simulink model "Detumbling_using_engine_sim"  (R2022b)
settings: Solver=VariableStepAuto  StartTime=0.0  StopTime=Params.tf  FixedStep=1e-2  RelTol=1e-8  AbsTol=1e-8
values from neighbouring files (symbols this model uses):
  Pitch_thrust_operator = abs(-1/( (1/(norm(Params.arm_vec1)))*(sin(gamma1)*sin(theta)*Params.arm_vec1(3)-cos(gamma1)*Params.arm_vec1(1))+         (1/(norm(Params.arm_vec2)))*(-sin(gamma2)*sin(theta)*Params.arm_vec2(3)-cos(gamma2)*Params.arm_vec2(1))+         (1/(norm(Params.arm_vec3)))*(sin(gamma3)*cos(theta)*Params.arm_vec3(3)+cos(gamma3)*Params.arm_vec3(2))+         (1/(norm(Params.arm_vec4)))*(sin(gamma4)*sin(theta)*Pa ...(+61 chars)    [Detumbling_using_engine_SimCode.m]
  Roll_thrust_operator = abs(-1/( (1/(norm(Params.arm_vec1)))*(-sin(gamma1)*cos(theta)*Params.arm_vec1(3)+cos(gamma1)*Params.arm_vec1(2))+         (1/(norm(Params.arm_vec2)))*(-sin(gamma2)*cos(theta)*Params.arm_vec2(3)+cos(gamma2)*Params.arm_vec2(2))+         (1/(norm(Params.arm_vec3)))*(sin(gamma3)*sin(theta)*Params.arm_vec3(3)-cos(gamma3)*Params.arm_vec3(1))+         (1/(norm(Params.arm_vec4)))*(sin(gamma4)*cos(theta)*P ...(+51 chars)    [Detumbling_using_engine_SimCode.m]
  tau_Thrusters = 30e-03    (= 0.03)    [Detumbling_using_engine_SimCode.m]
  w_c = [0,0,0]'    [Detumbling_using_engine_SimCode.m]
  Yaw_thrust_operator = abs(-1/( (1/(norm(Params.arm_vec1)))*(-sin(gamma1)*sin(theta)*Params.arm_vec1(2)+cos(theta)*sin(gamma1)*Params.arm_vec1(1))+         (1/(norm(Params.arm_vec2)))*(-sin(gamma2)*sin(theta)*Params.arm_vec2(2)-cos(theta)*sin(gamma2)*Params.arm_vec2(1))+         (1/(norm(Params.arm_vec3)))*(-sin(gamma3)*sin(theta)*Params.arm_vec3(2)-sin(gamma3)*cos(theta)*Params.arm_vec3(1))+         (1/(norm(Params.arm ...(+86 chars)    [Detumbling_using_engine_SimCode.m]
undefined symbols (not defined in the file or in its folder): gain, Params, Pitch, rad, Roll, s, T1, time_T1, Yaw
libraries: matrix_library x24, aerolibconvert2 x1, simulink_extras x1, sharedutil x1
(part 2 of 2)

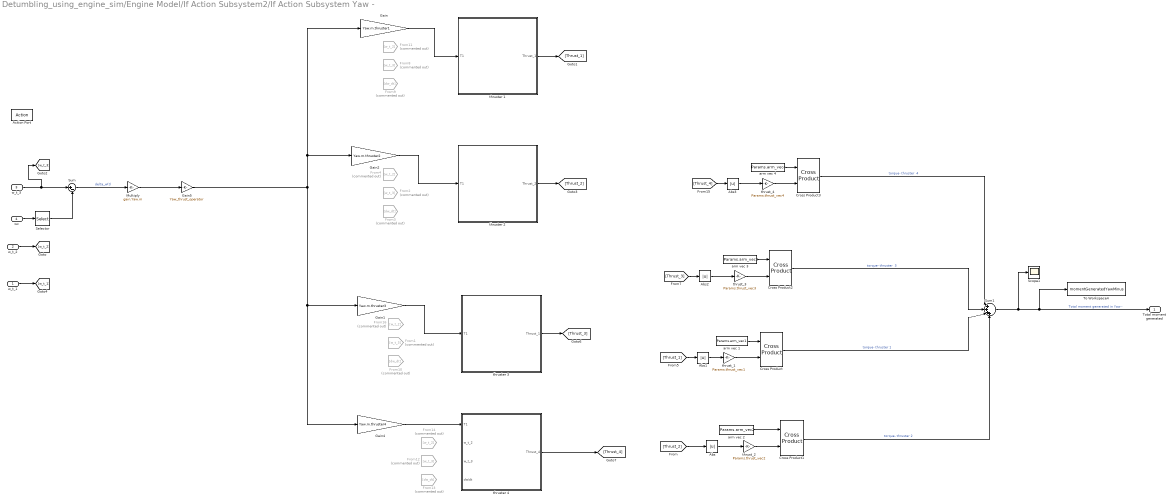
== system Detumbling_using_engine_sim/Engine Model/If Action Subsystem2/If Action Subsystem Yaw - ==
  w_t_1 : Inport
  w_t_2 : Inport  Port=2
  w_t_3 : Inport  Port=3
  wc : Inport  Port=4
  Action Port : ActionPort  ActionPortLabel=else
  Abs{,1..3} (4 alike) : Abs  SaturateOnIntegerOverflow=off
  Cross Product{,1..3} (4 alike) : matrix_library/Cross Product
  From{1..2,8,12} (4 alike) : From  Commented=on  GotoTag=w_t_3
  From{3,9..10,13} (4 alike) : From  Commented=on  GotoTag=dw_dt
  From{4,11,14,16} (4 alike) : From  Commented=on  GotoTag=w_t_2
  Gain : Gain  Gain=Yaw.m.thruster1
  Gain1 : Gain  Gain=Yaw.m.thruster3
  Gain2 : Gain  Gain=Yaw.m.thruster2
  Gain4 : Gain  Gain=Yaw.m.thruster4
  Gain5 : Gain  Gain=Yaw_thrust_operator
  Multiply : Gain  Gain=gain.Yaw.m
  Scope1 : Scope
  Selector : Selector  InputPortWidth=3  IndexOptions=Index vector (dialog)  Indices=3  OutputSizes=1
  Sum : Sum  Inputs=|+-
  Sum1 : Sum  Inputs=|++++
  To Workspace4 : ToWorkspace  VariableName=momentGeneratedYawMinus  SaveFormat=Timeseries  SampleTime=-1
  arm vec 1 : Constant  Value=Params.arm_vec1
  arm vec 2 : Constant  Value=Params.arm_vec2
  arm vec 3 : Constant  Value=Params.arm_vec3
  arm vec 4 : Constant  Value=Params.arm_vec4
  thrust_1 : Gain  Gain=Params.thrust_vec1
  thrust_2 : Gain  Gain=Params.thrust_vec2
  thrust_3 : Gain  Gain=Params.thrust_vec3
  thrust_4 : Gain  Gain=Params.thrust_vec4
  thruster 1 : Subsystem
  thruster 2 : Subsystem
  thruster 3 : Subsystem
  "thruster 4 " : Subsystem
  "Total moment generated " : Outport
  wires:
  w_t_1/1 -> [w_t_1]
  w_t_2/1 -> [w_t_2]
  w_t_3/1 -> [w_t_3], Sum/1
  wc/1 -> Selector/1
  Selector/1 -> Sum/2
  Multiply/1 -> Gain5/1
  thrust_3/1 -> Cross Product2/2
  Cross Product2/1 -> Sum1/2  "torque- thruster  3"
  Gain5/1 -> Gain2/1, Gain/1, Gain4/1, Gain1/1
  Cross Product3/1 -> Sum1/1  "torque- thruster  4"
  [Thrust_1] -> Abs1/1
  Gain/1 -> thruster 1/1(T1)
  Gain4/1 -> "thruster 4 "/1(T1)
  [Thrust_2] -> Abs/1
  arm vec 4/1 -> Cross Product3/1
  Cross Product/1 -> Sum1/3  "torque- thruster 1"
  thrust_4/1 -> Cross Product3/2
  arm vec 2/1 -> Cross Product1/1
  thruster 1/1(Thrust_1) -> [Thrust_1]
  arm vec 1/1 -> Cross Product/1
  thruster 3/1(Thrust_1) -> [Thrust_3]
  Cross Product1/1 -> Sum1/4  "torque- thruster 2"
  [Thrust_3] -> Abs2/1
  Gain2/1 -> thruster 2/1(T1)
  Sum/1 -> Multiply/1  "delta_w(t)"
  [Thrust_4] -> Abs3/1
  thrust_2/1 -> Cross Product1/2
  Abs1/1 -> thrust_1/1
  Sum1/1 -> Scope1/1, "Total moment generated "/1, To Workspace4/1  "Total moment generated in Yaw -"
  arm vec 3/1 -> Cross Product2/1
  Abs2/1 -> thrust_3/1
  "thruster 4 "/1(Thrust_4) -> [Thrust_4]
  Gain1/1 -> thruster 3/1(T1)
  Abs/1 -> thrust_2/1
  thruster 2/1(Thrust_2) -> [Thrust_2]
  Abs3/1 -> thrust_4/1
  thrust_1/1 -> Cross Product/2

== system Detumbling_using_engine_sim/Satellite Bus/Satellite Kinematics/CHI(q) ==
  q : Inport
  Demux : Demux
  Gain{1..6} (6 alike) : Gain  Gain=-1
  Vector Concatenate : Concatenate  NumInputs=4
  Vector Concatenate1 : Concatenate  NumInputs=4
  Vector Concatenate2 : Concatenate  NumInputs=4
  Vector Concatenate3 : Concatenate  NumInputs=3  Mode=Multidimensional array  ConcatenateDimension=2
  CHI : Outport
  wires:
  [q1] -> Vector Concatenate2/3
  [q3] -> Gain5/1
  Vector Concatenate3/1 -> CHI/1
  Vector Concatenate/1 -> Vector Concatenate3/1
  Vector Concatenate2/1 -> Vector Concatenate3/2
  q/1 -> Demux/1
  [q3] -> Gain3/1
  Gain3/1 -> Vector Concatenate2/1
  [q3] -> Vector Concatenate/2
  [q4] -> Vector Concatenate1/3
  [q1] -> Gain1/1
  Demux/2 -> [q2]
  Gain1/1 -> Vector Concatenate/4
  Demux/3 -> [q3]
  [q4] -> Vector Concatenate/1
  [q4] -> Vector Concatenate2/2
  Gain4/1 -> Vector Concatenate2/4
  [q2] -> Vector Concatenate1/1
  Demux/1 -> [q1]
  [q1] -> Gain6/1
  Gain6/1 -> Vector Concatenate1/2
  [q2] -> Gain2/1
  [q2] -> Gain4/1
  Gain2/1 -> Vector Concatenate/3
  Vector Concatenate1/1 -> Vector Concatenate3/3
  Demux/4 -> [q4]
  Gain5/1 -> Vector Concatenate1/4

== system Detumbling_using_engine_sim/Engine Model/If Action Subsystem/If Action Subsystem Roll +/thruster 1 ==
  T1 : Inport
  Abs : Abs  Commented=on  SaturateOnIntegerOverflow=off
  Clock : Clock  Commented=on
  Constant : Constant  Commented=on
  Divide : Product  Commented=on  Inputs=*/
  Divide1 : Product  Commented=on  Inputs=*/
  Divide2 : Product  Commented=on  Inputs=*/
  From{,1,3..4} (4 alike) : From  Commented=on  GotoTag=T1
  From2 : From  Commented=on  GotoTag=impulseBit_BiProp
  From5 : From  Commented=on  GotoTag=Stop_step
  Gain : Gain  Commented=on  Gain=Params.ImpulseBit_BiProp
  Goto2 : Goto  Commented=on  GotoTag=Stop_step
  Initial Body Angular rates [deg/sec] : Constant  Value=Params.ImpulseBit_BiProp
  Scope : Scope
  Step1 : Step  Commented=on  Time=Params.ImpulseBit_BiProp/T1  SampleTime=0
  Sum : Sum  Inputs=|+-
  Sum1 : Sum  Commented=on  Inputs=|++
  Switch : Switch  Commented=on  Criteria=u2 > Threshold  SaturateOnIntegerOverflow=off  InputSameDT=off
  "Time constant - open thruster " : TransferFcn  Denominator=[tau_Thrusters 1]
  To Workspace : ToWorkspace  Commented=on  VariableName=T1  SaveFormat=Timeseries  SampleTime=-1
  Variable Time Delay : VariableTransportDelay  Commented=on  MaximumDelay=50
  Thrust_1 : Outport
  wires:
  "Time constant - open thruster "/1 -> Sum/1
  Sum/1 -> Scope/1, Thrust_1/1
  Initial Body Angular rates [deg/sec]/1 -> [impulseBit_BiProp]
  Constant/1 -> Divide/1
  From/1 -> Divide/2
  Divide/1 -> Gain/1
  From1/1 -> Divide1/2
  Divide1/1 -> Sum1/2  "Requested Time [sec] The maximum possible"
  Clock/1 -> Sum1/1
  Sum1/1 -> Switch/2
  T1/1 -> [T1], To Workspace/1, "Time constant - open thruster "/1
  Divide2/1 -> Abs/1  "Maximum Time allowed"
  From2/1 -> Divide2/1
  From3/1 -> Divide2/2
  From4/1 -> Variable Time Delay/1
  Variable Time Delay/1 -> Goto2/1
  From5/1 -> Sum/2
  Abs/1 -> Variable Time Delay/2

== system Detumbling_using_engine_sim/Engine Model/If Action Subsystem/If Action Subsystem Roll +/thruster 2 ==
  T1 : Inport
  Abs : Abs  Commented=on  SaturateOnIntegerOverflow=off
  Divide2 : Product  Commented=on  Inputs=*/
  From2 : From  Commented=on  GotoTag=impulseBit_BiProp
  From3 : From  Commented=on  GotoTag=T2
  From4 : From  Commented=on  GotoTag=T2
  From5 : From  Commented=on  GotoTag=Stop_step
  Goto2 : Goto  Commented=on  GotoTag=Stop_step
  Initial Body Angular rates [deg/sec] : Constant  Value=Params.ImpulseBit_BiProp
  Scope : Scope
  Sum : Sum  Inputs=|+-
  "Time constant - open thruster " : TransferFcn  Denominator=[tau_Thrusters 1]
  To Workspace : ToWorkspace  Commented=on  VariableName=T1  SaveFormat=Timeseries  SampleTime=-1
  Variable Time Delay : VariableTransportDelay  Commented=on  MaximumDelay=50
  Thrust_2 : Outport
  wires:
  "Time constant - open thruster "/1 -> Sum/1
  Sum/1 -> Scope/1, Thrust_2/1
  Initial Body Angular rates [deg/sec]/1 -> [impulseBit_BiProp]
  T1/1 -> [T2], To Workspace/1, "Time constant - open thruster "/1
  From3/1 -> Divide2/2
  Divide2/1 -> Abs/1  "Maximum Time allowed"
  From4/1 -> Variable Time Delay/1
  Variable Time Delay/1 -> Goto2/1
  From2/1 -> Divide2/1
  From5/1 -> Sum/2
  Abs/1 -> Variable Time Delay/2

== system Detumbling_using_engine_sim/Engine Model/If Action Subsystem/If Action Subsystem Roll +/thruster 3 ==
  T1 : Inport
  Abs : Abs  Commented=on  SaturateOnIntegerOverflow=off
  Divide2 : Product  Commented=on  Inputs=*/
  From2 : From  Commented=on  GotoTag=impulseBit_BiProp
  From3 : From  Commented=on  GotoTag=T3
  From4 : From  Commented=on  GotoTag=T3
  From5 : From  Commented=on  GotoTag=Stop_step
  Goto2 : Goto  Commented=on  GotoTag=Stop_step
  Initial Body Angular rates [deg/sec] : Constant  Value=Params.ImpulseBit_BiProp
  Scope : Scope
  Sum : Sum  Inputs=|+-
  "Time constant - open thruster " : TransferFcn  Denominator=[tau_Thrusters 1]
  To Workspace : ToWorkspace  Commented=on  VariableName=T1  SaveFormat=Timeseries  SampleTime=-1
  Variable Time Delay1 : VariableTransportDelay  Commented=on  MaximumDelay=50
  Thrust_1 : Outport
  wires:
  "Time constant - open thruster "/1 -> Sum/1
  Sum/1 -> Scope/1, Thrust_1/1
  Initial Body Angular rates [deg/sec]/1 -> [impulseBit_BiProp]
  T1/1 -> [T3], To Workspace/1, "Time constant - open thruster "/1
  From3/1 -> Divide2/2
  Divide2/1 -> Abs/1  "Maximum Time allowed"
  From4/1 -> Variable Time Delay1/1
  Variable Time Delay1/1 -> Goto2/1
  From2/1 -> Divide2/1
  From5/1 -> Sum/2
  Abs/1 -> Variable Time Delay1/2

== system Detumbling_using_engine_sim/Engine Model/If Action Subsystem/If Action Subsystem Roll +/thruster 4  ==
  T1 : Inport
  w_t_2 : Inport  Port=2
  w_t_3 : Inport  Port=3
  dw/dt : Inport  Port=4
  Abs : Abs  Commented=on  SaturateOnIntegerOverflow=off
  Divide2 : Product  Commented=on  Inputs=*/
  From2 : From  Commented=on  GotoTag=impulseBit_BiProp
  From3 : From  Commented=on  GotoTag=T1
  From4 : From  Commented=on  GotoTag=T1
  From5 : From  Commented=on  GotoTag=Stop_step
  Goto2 : Goto  Commented=on  GotoTag=Stop_step
  Initial Body Angular rates [deg/sec] : Constant  Value=Params.ImpulseBit_BiProp
  Sum : Sum  Inputs=|+-
  "Time constant - open thruster " : TransferFcn  Denominator=[tau_Thrusters 1]
  To Workspace : ToWorkspace  Commented=on  VariableName=T1  SaveFormat=Timeseries  SampleTime=-1
  Variable Time Delay1 : VariableTransportDelay  Commented=on  MaximumDelay=50
  Thrust_4 : Outport
  wires:
  "Time constant - open thruster "/1 -> Sum/1
  Sum/1 -> Thrust_4/1
  Initial Body Angular rates [deg/sec]/1 -> [impulseBit_BiProp]
  T1/1 -> [T1], To Workspace/1, "Time constant - open thruster "/1
  From2/1 -> Divide2/1
  From3/1 -> Divide2/2
  Divide2/1 -> Abs/1  "Maximum Time allowed"
  From4/1 -> Variable Time Delay1/1
  Variable Time Delay1/1 -> Goto2/1
  From5/1 -> Sum/2
  Abs/1 -> Variable Time Delay1/2

== system Detumbling_using_engine_sim/Engine Model/If Action Subsystem/If Action Subsystem Roll -/thruster 1 ==
  T1 : Inport
  Abs : Abs  Commented=on  SaturateOnIntegerOverflow=off
  Clock : Clock  Commented=on
  Constant : Constant  Commented=on
  Divide : Product  Commented=on  Inputs=*/
  Divide1 : Product  Commented=on  Inputs=*/
  Divide2 : Product  Commented=on  Inputs=*/
  From{,1,3..4} (4 alike) : From  Commented=on  GotoTag=T1
  From2 : From  Commented=on  GotoTag=impulseBit_BiProp
  From5 : From  Commented=on  GotoTag=Stop_step
  Gain : Gain  Commented=on  Gain=Params.ImpulseBit_BiProp
  Goto2 : Goto  Commented=on  GotoTag=Stop_step
  Initial Body Angular rates [deg/sec] : Constant  Value=Params.ImpulseBit_BiProp
  Scope : Scope
  Step1 : Step  Commented=on  Time=Params.ImpulseBit_BiProp/T1  SampleTime=0
  Sum : Sum  Inputs=|+-
  Sum1 : Sum  Commented=on  Inputs=|++
  Switch : Switch  Commented=on  Criteria=u2 > Threshold  SaturateOnIntegerOverflow=off  InputSameDT=off
  "Time constant - open thruster " : TransferFcn  Denominator=[tau_Thrusters 1]
  To Workspace : ToWorkspace  Commented=on  VariableName=T1  SaveFormat=Timeseries  SampleTime=-1
  Variable Time Delay : VariableTransportDelay  Commented=on  MaximumDelay=50
  Thrust_1 : Outport
  wires:
  "Time constant - open thruster "/1 -> Sum/1
  Sum/1 -> Scope/1, Thrust_1/1
  Initial Body Angular rates [deg/sec]/1 -> [impulseBit_BiProp]
  Constant/1 -> Divide/1
  From/1 -> Divide/2
  Divide/1 -> Gain/1
  From1/1 -> Divide1/2
  Divide1/1 -> Sum1/2  "Requested Time [sec] The maximum possible"
  Clock/1 -> Sum1/1
  Sum1/1 -> Switch/2
  T1/1 -> [T1], To Workspace/1, "Time constant - open thruster "/1
  Divide2/1 -> Abs/1  "Maximum Time allowed"
  From2/1 -> Divide2/1
  From3/1 -> Divide2/2
  From4/1 -> Variable Time Delay/1
  Variable Time Delay/1 -> Goto2/1
  From5/1 -> Sum/2
  Abs/1 -> Variable Time Delay/2

== system Detumbling_using_engine_sim/Engine Model/If Action Subsystem/If Action Subsystem Roll -/thruster 2 ==
  T1 : Inport
  Abs : Abs  Commented=on  SaturateOnIntegerOverflow=off
  Divide2 : Product  Commented=on  Inputs=*/
  From2 : From  Commented=on  GotoTag=impulseBit_BiProp
  From3 : From  Commented=on  GotoTag=T2
  From4 : From  Commented=on  GotoTag=T2
  From5 : From  Commented=on  GotoTag=Stop_step
  Goto2 : Goto  Commented=on  GotoTag=Stop_step
  Initial Body Angular rates [deg/sec] : Constant  Value=Params.ImpulseBit_BiProp
  Scope : Scope
  Sum : Sum  Inputs=|+-
  "Time constant - open thruster " : TransferFcn  Denominator=[tau_Thrusters 1]
  To Workspace : ToWorkspace  Commented=on  VariableName=T1  SaveFormat=Timeseries  SampleTime=-1
  Variable Time Delay : VariableTransportDelay  Commented=on  MaximumDelay=50
  Thrust_2 : Outport
  wires:
  "Time constant - open thruster "/1 -> Sum/1
  Sum/1 -> Scope/1, Thrust_2/1
  Initial Body Angular rates [deg/sec]/1 -> [impulseBit_BiProp]
  T1/1 -> [T2], To Workspace/1, "Time constant - open thruster "/1
  From3/1 -> Divide2/2
  Divide2/1 -> Abs/1  "Maximum Time allowed"
  From4/1 -> Variable Time Delay/1
  Variable Time Delay/1 -> Goto2/1
  From2/1 -> Divide2/1
  From5/1 -> Sum/2
  Abs/1 -> Variable Time Delay/2

== system Detumbling_using_engine_sim/Engine Model/If Action Subsystem/If Action Subsystem Roll -/thruster 3 ==
  T1 : Inport
  Abs : Abs  Commented=on  SaturateOnIntegerOverflow=off
  Divide2 : Product  Commented=on  Inputs=*/
  From2 : From  Commented=on  GotoTag=impulseBit_BiProp
  From3 : From  Commented=on  GotoTag=T3
  From4 : From  Commented=on  GotoTag=T3
  From5 : From  Commented=on  GotoTag=Stop_step
  Goto2 : Goto  Commented=on  GotoTag=Stop_step
  Initial Body Angular rates [deg/sec] : Constant  Value=Params.ImpulseBit_BiProp
  Scope : Scope
  Sum : Sum  Inputs=|+-
  "Time constant - open thruster " : TransferFcn  Denominator=[tau_Thrusters 1]
  To Workspace : ToWorkspace  Commented=on  VariableName=T1  SaveFormat=Timeseries  SampleTime=-1
  Variable Time Delay1 : VariableTransportDelay  Commented=on  MaximumDelay=50
  Thrust_1 : Outport
  wires:
  "Time constant - open thruster "/1 -> Sum/1
  Sum/1 -> Scope/1, Thrust_1/1
  Initial Body Angular rates [deg/sec]/1 -> [impulseBit_BiProp]
  T1/1 -> [T3], To Workspace/1, "Time constant - open thruster "/1
  From3/1 -> Divide2/2
  Divide2/1 -> Abs/1  "Maximum Time allowed"
  From4/1 -> Variable Time Delay1/1
  Variable Time Delay1/1 -> Goto2/1
  From2/1 -> Divide2/1
  From5/1 -> Sum/2
  Abs/1 -> Variable Time Delay1/2

== system Detumbling_using_engine_sim/Engine Model/If Action Subsystem/If Action Subsystem Roll -/thruster 4  ==
  T1 : Inport
  w_t_2 : Inport  Port=2
  w_t_3 : Inport  Port=3
  dw/dt : Inport  Port=4
  Abs : Abs  Commented=on  SaturateOnIntegerOverflow=off
  Divide2 : Product  Commented=on  Inputs=*/
  From2 : From  Commented=on  GotoTag=impulseBit_BiProp
  From3 : From  Commented=on  GotoTag=T1
  From4 : From  Commented=on  GotoTag=T1
  From5 : From  Commented=on  GotoTag=Stop_step
  Goto2 : Goto  Commented=on  GotoTag=Stop_step
  Initial Body Angular rates [deg/sec] : Constant  Value=Params.ImpulseBit_BiProp
  Sum : Sum  Inputs=|+-
  "Time constant - open thruster " : TransferFcn  Denominator=[tau_Thrusters 1]
  To Workspace : ToWorkspace  Commented=on  VariableName=T1  SaveFormat=Timeseries  SampleTime=-1
  Variable Time Delay1 : VariableTransportDelay  Commented=on  MaximumDelay=50
  Thrust_4 : Outport
  wires:
  "Time constant - open thruster "/1 -> Sum/1
  Sum/1 -> Thrust_4/1
  Initial Body Angular rates [deg/sec]/1 -> [impulseBit_BiProp]
  T1/1 -> [T1], To Workspace/1, "Time constant - open thruster "/1
  From2/1 -> Divide2/1
  From3/1 -> Divide2/2
  Divide2/1 -> Abs/1  "Maximum Time allowed"
  From4/1 -> Variable Time Delay1/1
  Variable Time Delay1/1 -> Goto2/1
  From5/1 -> Sum/2
  Abs/1 -> Variable Time Delay1/2

== system Detumbling_using_engine_sim/Engine Model/If Action Subsystem1/If Action Subsystem Pitch +/thruster 1 ==
  T1 : Inport
  Abs : Abs  Commented=on  SaturateOnIntegerOverflow=off
  Clock : Clock  Commented=on
  Constant : Constant  Commented=on
  Divide : Product  Commented=on  Inputs=*/
  Divide1 : Product  Commented=on  Inputs=*/
  Divide2 : Product  Commented=on  Inputs=*/
  From{,1,3..4} (4 alike) : From  Commented=on  GotoTag=T1
  From2 : From  Commented=on  GotoTag=impulseBit_BiProp
  From5 : From  Commented=on  GotoTag=Stop_step
  Gain : Gain  Commented=on  Gain=Params.ImpulseBit_BiProp
  Goto2 : Goto  Commented=on  GotoTag=Stop_step
  Initial Body Angular rates [deg/sec] : Constant  Value=Params.ImpulseBit_BiProp
  Scope : Scope
  Step1 : Step  Commented=on  Time=Params.ImpulseBit_BiProp/T1  SampleTime=0
  Sum : Sum  Inputs=|+-
  Sum1 : Sum  Commented=on  Inputs=|++
  Switch : Switch  Commented=on  Criteria=u2 > Threshold  SaturateOnIntegerOverflow=off  InputSameDT=off
  "Time constant - open thruster " : TransferFcn  Denominator=[tau_Thrusters 1]
  To Workspace : ToWorkspace  Commented=on  VariableName=T1  SaveFormat=Timeseries  SampleTime=-1
  Variable Time Delay : VariableTransportDelay  Commented=on  MaximumDelay=50
  Thrust_1 : Outport
  wires:
  "Time constant - open thruster "/1 -> Sum/1
  Sum/1 -> Scope/1, Thrust_1/1
  Initial Body Angular rates [deg/sec]/1 -> [impulseBit_BiProp]
  Constant/1 -> Divide/1
  From/1 -> Divide/2
  Divide/1 -> Gain/1
  From1/1 -> Divide1/2
  Divide1/1 -> Sum1/2  "Requested Time [sec] The maximum possible"
  Clock/1 -> Sum1/1
  Sum1/1 -> Switch/2
  T1/1 -> [T1], To Workspace/1, "Time constant - open thruster "/1
  Divide2/1 -> Abs/1  "Maximum Time allowed"
  From2/1 -> Divide2/1
  From3/1 -> Divide2/2
  From4/1 -> Variable Time Delay/1
  Variable Time Delay/1 -> Goto2/1
  From5/1 -> Sum/2
  Abs/1 -> Variable Time Delay/2

== system Detumbling_using_engine_sim/Engine Model/If Action Subsystem1/If Action Subsystem Pitch +/thruster 2 ==
  T1 : Inport
  Abs : Abs  Commented=on  SaturateOnIntegerOverflow=off
  Divide2 : Product  Commented=on  Inputs=*/
  From2 : From  Commented=on  GotoTag=impulseBit_BiProp
  From3 : From  Commented=on  GotoTag=T2
  From4 : From  Commented=on  GotoTag=T2
  From5 : From  Commented=on  GotoTag=Stop_step
  Goto2 : Goto  Commented=on  GotoTag=Stop_step
  Initial Body Angular rates [deg/sec] : Constant  Value=Params.ImpulseBit_BiProp
  Scope : Scope
  Sum : Sum  Inputs=|+-
  "Time constant - open thruster " : TransferFcn  Denominator=[tau_Thrusters 1]
  To Workspace : ToWorkspace  Commented=on  VariableName=T1  SaveFormat=Timeseries  SampleTime=-1
  Variable Time Delay : VariableTransportDelay  Commented=on  MaximumDelay=50
  Thrust_2 : Outport
  wires:
  "Time constant - open thruster "/1 -> Sum/1
  Sum/1 -> Scope/1, Thrust_2/1
  Initial Body Angular rates [deg/sec]/1 -> [impulseBit_BiProp]
  T1/1 -> [T2], To Workspace/1, "Time constant - open thruster "/1
  From3/1 -> Divide2/2
  Divide2/1 -> Abs/1  "Maximum Time allowed"
  From4/1 -> Variable Time Delay/1
  Variable Time Delay/1 -> Goto2/1
  From2/1 -> Divide2/1
  From5/1 -> Sum/2
  Abs/1 -> Variable Time Delay/2

== system Detumbling_using_engine_sim/Engine Model/If Action Subsystem1/If Action Subsystem Pitch +/thruster 3 ==
  T1 : Inport
  Abs : Abs  Commented=on  SaturateOnIntegerOverflow=off
  Divide2 : Product  Commented=on  Inputs=*/
  From2 : From  Commented=on  GotoTag=impulseBit_BiProp
  From3 : From  Commented=on  GotoTag=T3
  From4 : From  Commented=on  GotoTag=T3
  From5 : From  Commented=on  GotoTag=Stop_step
  Goto2 : Goto  Commented=on  GotoTag=Stop_step
  Initial Body Angular rates [deg/sec] : Constant  Value=Params.ImpulseBit_BiProp
  Scope : Scope
  Sum : Sum  Inputs=|+-
  "Time constant - open thruster " : TransferFcn  Denominator=[tau_Thrusters 1]
  To Workspace : ToWorkspace  Commented=on  VariableName=T1  SaveFormat=Timeseries  SampleTime=-1
  Variable Time Delay1 : VariableTransportDelay  Commented=on  MaximumDelay=50
  Thrust_1 : Outport
  wires:
  "Time constant - open thruster "/1 -> Sum/1
  Sum/1 -> Scope/1, Thrust_1/1
  Initial Body Angular rates [deg/sec]/1 -> [impulseBit_BiProp]
  T1/1 -> [T3], To Workspace/1, "Time constant - open thruster "/1
  From3/1 -> Divide2/2
  Divide2/1 -> Abs/1  "Maximum Time allowed"
  From4/1 -> Variable Time Delay1/1
  Variable Time Delay1/1 -> Goto2/1
  From2/1 -> Divide2/1
  From5/1 -> Sum/2
  Abs/1 -> Variable Time Delay1/2

== system Detumbling_using_engine_sim/Engine Model/If Action Subsystem1/If Action Subsystem Pitch +/thruster 4  ==
  T1 : Inport
  w_t_2 : Inport  Port=2
  w_t_3 : Inport  Port=3
  dw/dt : Inport  Port=4
  Abs : Abs  Commented=on  SaturateOnIntegerOverflow=off
  Divide2 : Product  Commented=on  Inputs=*/
  From2 : From  Commented=on  GotoTag=impulseBit_BiProp
  From3 : From  Commented=on  GotoTag=T1
  From4 : From  Commented=on  GotoTag=T1
  From5 : From  Commented=on  GotoTag=Stop_step
  Goto2 : Goto  Commented=on  GotoTag=Stop_step
  Initial Body Angular rates [deg/sec] : Constant  Value=Params.ImpulseBit_BiProp
  Sum : Sum  Inputs=|+-
  "Time constant - open thruster " : TransferFcn  Denominator=[tau_Thrusters 1]
  To Workspace : ToWorkspace  Commented=on  VariableName=T1  SaveFormat=Timeseries  SampleTime=-1
  Variable Time Delay1 : VariableTransportDelay  Commented=on  MaximumDelay=50
  Thrust_4 : Outport
  wires:
  "Time constant - open thruster "/1 -> Sum/1
  Sum/1 -> Thrust_4/1
  Initial Body Angular rates [deg/sec]/1 -> [impulseBit_BiProp]
  T1/1 -> [T1], To Workspace/1, "Time constant - open thruster "/1
  From2/1 -> Divide2/1
  From3/1 -> Divide2/2
  Divide2/1 -> Abs/1  "Maximum Time allowed"
  From4/1 -> Variable Time Delay1/1
  Variable Time Delay1/1 -> Goto2/1
  From5/1 -> Sum/2
  Abs/1 -> Variable Time Delay1/2

== system Detumbling_using_engine_sim/Engine Model/If Action Subsystem1/If Action Subsystem Pitch -/thruster 1 ==
  T1 : Inport
  Abs : Abs  Commented=on  SaturateOnIntegerOverflow=off
  Clock : Clock  Commented=on
  Constant : Constant  Commented=on
  Divide : Product  Commented=on  Inputs=*/
  Divide1 : Product  Commented=on  Inputs=*/
  Divide2 : Product  Commented=on  Inputs=*/
  From{,1,3..4} (4 alike) : From  Commented=on  GotoTag=T1
  From2 : From  Commented=on  GotoTag=impulseBit_BiProp
  From5 : From  Commented=on  GotoTag=Stop_step
  Gain : Gain  Commented=on  Gain=Params.ImpulseBit_BiProp
  Goto2 : Goto  Commented=on  GotoTag=Stop_step
  Initial Body Angular rates [deg/sec] : Constant  Value=Params.ImpulseBit_BiProp
  Scope : Scope
  Step1 : Step  Commented=on  Time=Params.ImpulseBit_BiProp/T1  SampleTime=0
  Sum : Sum  Inputs=|+-
  Sum1 : Sum  Commented=on  Inputs=|++
  Switch : Switch  Commented=on  Criteria=u2 > Threshold  SaturateOnIntegerOverflow=off  InputSameDT=off
  "Time constant - open thruster " : TransferFcn  Denominator=[tau_Thrusters 1]
  To Workspace : ToWorkspace  Commented=on  VariableName=T1  SaveFormat=Timeseries  SampleTime=-1
  Variable Time Delay : VariableTransportDelay  Commented=on  MaximumDelay=50
  Thrust_1 : Outport
  wires:
  "Time constant - open thruster "/1 -> Sum/1
  Sum/1 -> Scope/1, Thrust_1/1
  Initial Body Angular rates [deg/sec]/1 -> [impulseBit_BiProp]
  Constant/1 -> Divide/1
  From/1 -> Divide/2
  Divide/1 -> Gain/1
  From1/1 -> Divide1/2
  Divide1/1 -> Sum1/2  "Requested Time [sec] The maximum possible"
  Clock/1 -> Sum1/1
  Sum1/1 -> Switch/2
  T1/1 -> [T1], To Workspace/1, "Time constant - open thruster "/1
  Divide2/1 -> Abs/1  "Maximum Time allowed"
  From2/1 -> Divide2/1
  From3/1 -> Divide2/2
  From4/1 -> Variable Time Delay/1
  Variable Time Delay/1 -> Goto2/1
  From5/1 -> Sum/2
  Abs/1 -> Variable Time Delay/2

== system Detumbling_using_engine_sim/Engine Model/If Action Subsystem1/If Action Subsystem Pitch -/thruster 2 ==
  T1 : Inport
  Abs : Abs  Commented=on  SaturateOnIntegerOverflow=off
  Divide2 : Product  Commented=on  Inputs=*/
  From2 : From  Commented=on  GotoTag=impulseBit_BiProp
  From3 : From  Commented=on  GotoTag=T2
  From4 : From  Commented=on  GotoTag=T2
  From5 : From  Commented=on  GotoTag=Stop_step
  Goto2 : Goto  Commented=on  GotoTag=Stop_step
  Initial Body Angular rates [deg/sec] : Constant  Value=Params.ImpulseBit_BiProp
  Scope : Scope
  Sum : Sum  Inputs=|+-
  "Time constant - open thruster " : TransferFcn  Denominator=[tau_Thrusters 1]
  To Workspace : ToWorkspace  Commented=on  VariableName=T1  SaveFormat=Timeseries  SampleTime=-1
  Variable Time Delay : VariableTransportDelay  Commented=on  MaximumDelay=50
  Thrust_2 : Outport
  wires:
  "Time constant - open thruster "/1 -> Sum/1
  Sum/1 -> Scope/1, Thrust_2/1
  Initial Body Angular rates [deg/sec]/1 -> [impulseBit_BiProp]
  T1/1 -> [T2], To Workspace/1, "Time constant - open thruster "/1
  From3/1 -> Divide2/2
  Divide2/1 -> Abs/1  "Maximum Time allowed"
  From4/1 -> Variable Time Delay/1
  Variable Time Delay/1 -> Goto2/1
  From2/1 -> Divide2/1
  From5/1 -> Sum/2
  Abs/1 -> Variable Time Delay/2

== system Detumbling_using_engine_sim/Engine Model/If Action Subsystem1/If Action Subsystem Pitch -/thruster 3 ==
  T1 : Inport
  Abs : Abs  Commented=on  SaturateOnIntegerOverflow=off
  Divide2 : Product  Commented=on  Inputs=*/
  From2 : From  Commented=on  GotoTag=impulseBit_BiProp
  From3 : From  Commented=on  GotoTag=T3
  From4 : From  Commented=on  GotoTag=T3
  From5 : From  Commented=on  GotoTag=Stop_step
  Goto2 : Goto  Commented=on  GotoTag=Stop_step
  Initial Body Angular rates [deg/sec] : Constant  Value=Params.ImpulseBit_BiProp
  Scope : Scope
  Sum : Sum  Inputs=|+-
  "Time constant - open thruster " : TransferFcn  Denominator=[tau_Thrusters 1]
  To Workspace : ToWorkspace  Commented=on  VariableName=T1  SaveFormat=Timeseries  SampleTime=-1
  Variable Time Delay1 : VariableTransportDelay  Commented=on  MaximumDelay=50
  Thrust_1 : Outport
  wires:
  "Time constant - open thruster "/1 -> Sum/1
  Sum/1 -> Scope/1, Thrust_1/1
  Initial Body Angular rates [deg/sec]/1 -> [impulseBit_BiProp]
  T1/1 -> [T3], To Workspace/1, "Time constant - open thruster "/1
  From3/1 -> Divide2/2
  Divide2/1 -> Abs/1  "Maximum Time allowed"
  From4/1 -> Variable Time Delay1/1
  Variable Time Delay1/1 -> Goto2/1
  From2/1 -> Divide2/1
  From5/1 -> Sum/2
  Abs/1 -> Variable Time Delay1/2

== system Detumbling_using_engine_sim/Engine Model/If Action Subsystem1/If Action Subsystem Pitch -/thruster 4  ==
  T1 : Inport
  w_t_2 : Inport  Port=2
  w_t_3 : Inport  Port=3
  dw/dt : Inport  Port=4
  Abs : Abs  Commented=on  SaturateOnIntegerOverflow=off
  Divide2 : Product  Commented=on  Inputs=*/
  From2 : From  Commented=on  GotoTag=impulseBit_BiProp
  From3 : From  Commented=on  GotoTag=T1
  From4 : From  Commented=on  GotoTag=T1
  From5 : From  Commented=on  GotoTag=Stop_step
  Goto2 : Goto  Commented=on  GotoTag=Stop_step
  Initial Body Angular rates [deg/sec] : Constant  Value=Params.ImpulseBit_BiProp
  Sum : Sum  Inputs=|+-
  "Time constant - open thruster " : TransferFcn  Denominator=[tau_Thrusters 1]
  To Workspace : ToWorkspace  Commented=on  VariableName=T1  SaveFormat=Timeseries  SampleTime=-1
  Variable Time Delay1 : VariableTransportDelay  Commented=on  MaximumDelay=50
  Thrust_4 : Outport
  wires:
  "Time constant - open thruster "/1 -> Sum/1
  Sum/1 -> Thrust_4/1
  Initial Body Angular rates [deg/sec]/1 -> [impulseBit_BiProp]
  T1/1 -> [T1], To Workspace/1, "Time constant - open thruster "/1
  From2/1 -> Divide2/1
  From3/1 -> Divide2/2
  Divide2/1 -> Abs/1  "Maximum Time allowed"
  From4/1 -> Variable Time Delay1/1
  Variable Time Delay1/1 -> Goto2/1
  From5/1 -> Sum/2
  Abs/1 -> Variable Time Delay1/2

== system Detumbling_using_engine_sim/Engine Model/If Action Subsystem2/If Action Subsystem Yaw +/thruster 1 ==
  T1 : Inport
  Abs : Abs  Commented=on  SaturateOnIntegerOverflow=off
  Clock : Clock  Commented=on
  Constant : Constant  Commented=on
  Divide : Product  Commented=on  Inputs=*/
  Divide1 : Product  Commented=on  Inputs=*/
  Divide2 : Product  Commented=on  Inputs=*/
  From{,1,3..4} (4 alike) : From  Commented=on  GotoTag=T1
  From2 : From  Commented=on  GotoTag=impulseBit_BiProp
  From5 : From  Commented=on  GotoTag=Stop_step
  Gain : Gain  Commented=on  Gain=Params.ImpulseBit_BiProp
  Goto2 : Goto  Commented=on  GotoTag=Stop_step
  Initial Body Angular rates [deg/sec] : Constant  Value=Params.ImpulseBit_BiProp
  Scope : Scope
  Step1 : Step  Commented=on  Time=Params.ImpulseBit_BiProp/T1  SampleTime=0
  Sum : Sum  Inputs=|+-
  Sum1 : Sum  Commented=on  Inputs=|++
  Switch : Switch  Commented=on  Criteria=u2 > Threshold  SaturateOnIntegerOverflow=off  InputSameDT=off
  "Time constant - open thruster " : TransferFcn  Denominator=[tau_Thrusters 1]
  To Workspace : ToWorkspace  Commented=on  VariableName=T1  SaveFormat=Timeseries  SampleTime=-1
  Variable Time Delay : VariableTransportDelay  Commented=on  MaximumDelay=50
  Thrust_1 : Outport
  wires:
  "Time constant - open thruster "/1 -> Sum/1
  Sum/1 -> Scope/1, Thrust_1/1
  Initial Body Angular rates [deg/sec]/1 -> [impulseBit_BiProp]
  Constant/1 -> Divide/1
  From/1 -> Divide/2
  Divide/1 -> Gain/1
  From1/1 -> Divide1/2
  Divide1/1 -> Sum1/2  "Requested Time [sec] The maximum possible"
  Clock/1 -> Sum1/1
  Sum1/1 -> Switch/2
  T1/1 -> [T1], To Workspace/1, "Time constant - open thruster "/1
  Divide2/1 -> Abs/1  "Maximum Time allowed"
  From2/1 -> Divide2/1
  From3/1 -> Divide2/2
  From4/1 -> Variable Time Delay/1
  Variable Time Delay/1 -> Goto2/1
  From5/1 -> Sum/2
  Abs/1 -> Variable Time Delay/2

== system Detumbling_using_engine_sim/Engine Model/If Action Subsystem2/If Action Subsystem Yaw +/thruster 2 ==
  T1 : Inport
  Abs : Abs  Commented=on  SaturateOnIntegerOverflow=off
  Divide2 : Product  Commented=on  Inputs=*/
  From2 : From  Commented=on  GotoTag=impulseBit_BiProp
  From3 : From  Commented=on  GotoTag=T2
  From4 : From  Commented=on  GotoTag=T2
  From5 : From  Commented=on  GotoTag=Stop_step
  Goto2 : Goto  Commented=on  GotoTag=Stop_step
  Initial Body Angular rates [deg/sec] : Constant  Value=Params.ImpulseBit_BiProp
  Scope : Scope
  Sum : Sum  Inputs=|+-
  "Time constant - open thruster " : TransferFcn  Denominator=[tau_Thrusters 1]
  To Workspace : ToWorkspace  Commented=on  VariableName=T1  SaveFormat=Timeseries  SampleTime=-1
  Variable Time Delay : VariableTransportDelay  Commented=on  MaximumDelay=50
  Thrust_2 : Outport
  wires:
  "Time constant - open thruster "/1 -> Sum/1
  Sum/1 -> Scope/1, Thrust_2/1
  Initial Body Angular rates [deg/sec]/1 -> [impulseBit_BiProp]
  T1/1 -> [T2], To Workspace/1, "Time constant - open thruster "/1
  From3/1 -> Divide2/2
  Divide2/1 -> Abs/1  "Maximum Time allowed"
  From4/1 -> Variable Time Delay/1
  Variable Time Delay/1 -> Goto2/1
  From2/1 -> Divide2/1
  From5/1 -> Sum/2
  Abs/1 -> Variable Time Delay/2

== system Detumbling_using_engine_sim/Engine Model/If Action Subsystem2/If Action Subsystem Yaw +/thruster 3 ==
  T1 : Inport
  Abs : Abs  Commented=on  SaturateOnIntegerOverflow=off
  Divide2 : Product  Commented=on  Inputs=*/
  From2 : From  Commented=on  GotoTag=impulseBit_BiProp
  From3 : From  Commented=on  GotoTag=T3
  From4 : From  Commented=on  GotoTag=T3
  From5 : From  Commented=on  GotoTag=Stop_step
  Goto2 : Goto  Commented=on  GotoTag=Stop_step
  Initial Body Angular rates [deg/sec] : Constant  Value=Params.ImpulseBit_BiProp
  Scope : Scope
  Sum : Sum  Inputs=|+-
  "Time constant - open thruster " : TransferFcn  Denominator=[tau_Thrusters 1]
  To Workspace : ToWorkspace  Commented=on  VariableName=T1  SaveFormat=Timeseries  SampleTime=-1
  Variable Time Delay1 : VariableTransportDelay  Commented=on  MaximumDelay=50
  Thrust_1 : Outport
  wires:
  "Time constant - open thruster "/1 -> Sum/1
  Sum/1 -> Scope/1, Thrust_1/1
  Initial Body Angular rates [deg/sec]/1 -> [impulseBit_BiProp]
  T1/1 -> [T3], To Workspace/1, "Time constant - open thruster "/1
  From3/1 -> Divide2/2
  Divide2/1 -> Abs/1  "Maximum Time allowed"
  From4/1 -> Variable Time Delay1/1
  Variable Time Delay1/1 -> Goto2/1
  From2/1 -> Divide2/1
  From5/1 -> Sum/2
  Abs/1 -> Variable Time Delay1/2

== system Detumbling_using_engine_sim/Engine Model/If Action Subsystem2/If Action Subsystem Yaw +/thruster 4  ==
  T1 : Inport
  w_t_2 : Inport  Port=2
  w_t_3 : Inport  Port=3
  dw/dt : Inport  Port=4
  Abs : Abs  Commented=on  SaturateOnIntegerOverflow=off
  Divide2 : Product  Commented=on  Inputs=*/
  From2 : From  Commented=on  GotoTag=impulseBit_BiProp
  From3 : From  Commented=on  GotoTag=T1
  From4 : From  Commented=on  GotoTag=T1
  From5 : From  Commented=on  GotoTag=Stop_step
  Goto2 : Goto  Commented=on  GotoTag=Stop_step
  Initial Body Angular rates [deg/sec] : Constant  Value=Params.ImpulseBit_BiProp
  Sum : Sum  Inputs=|+-
  "Time constant - open thruster " : TransferFcn  Denominator=[tau_Thrusters 1]
  To Workspace : ToWorkspace  Commented=on  VariableName=T1  SaveFormat=Timeseries  SampleTime=-1
  Variable Time Delay1 : VariableTransportDelay  Commented=on  MaximumDelay=50
  Thrust_4 : Outport
  wires:
  "Time constant - open thruster "/1 -> Sum/1
  Sum/1 -> Thrust_4/1
  Initial Body Angular rates [deg/sec]/1 -> [impulseBit_BiProp]
  T1/1 -> [T1], To Workspace/1, "Time constant - open thruster "/1
  From2/1 -> Divide2/1
  From3/1 -> Divide2/2
  Divide2/1 -> Abs/1  "Maximum Time allowed"
  From4/1 -> Variable Time Delay1/1
  Variable Time Delay1/1 -> Goto2/1
  From5/1 -> Sum/2
  Abs/1 -> Variable Time Delay1/2

== system Detumbling_using_engine_sim/Engine Model/If Action Subsystem2/If Action Subsystem Yaw -/thruster 1 ==
  T1 : Inport
  Abs : Abs  Commented=on  SaturateOnIntegerOverflow=off
  Clock : Clock  Commented=on
  Constant : Constant  Commented=on
  Divide : Product  Commented=on  Inputs=*/
  Divide1 : Product  Commented=on  Inputs=*/
  Divide2 : Product  Commented=on  Inputs=*/
  From{,1,3..4} (4 alike) : From  Commented=on  GotoTag=T1
  From2 : From  Commented=on  GotoTag=impulseBit_BiProp
  From5 : From  Commented=on  GotoTag=Stop_step
  Gain : Gain  Commented=on  Gain=Params.ImpulseBit_BiProp
  Goto2 : Goto  Commented=on  GotoTag=Stop_step
  Initial Body Angular rates [deg/sec] : Constant  Value=Params.ImpulseBit_BiProp
  Scope : Scope
  Step1 : Step  Commented=on  Time=Params.ImpulseBit_BiProp/T1  SampleTime=0
  Sum : Sum  Inputs=|+-
  Sum1 : Sum  Commented=on  Inputs=|++
  Switch : Switch  Commented=on  Criteria=u2 > Threshold  SaturateOnIntegerOverflow=off  InputSameDT=off
  "Time constant - open thruster " : TransferFcn  Denominator=[tau_Thrusters 1]
  To Workspace : ToWorkspace  Commented=on  VariableName=T1  SaveFormat=Timeseries  SampleTime=-1
  Variable Time Delay : VariableTransportDelay  Commented=on  MaximumDelay=50
  Thrust_1 : Outport
  wires:
  "Time constant - open thruster "/1 -> Sum/1
  Sum/1 -> Scope/1, Thrust_1/1
  Initial Body Angular rates [deg/sec]/1 -> [impulseBit_BiProp]
  Constant/1 -> Divide/1
  From/1 -> Divide/2
  Divide/1 -> Gain/1
  From1/1 -> Divide1/2
  Divide1/1 -> Sum1/2  "Requested Time [sec] The maximum possible"
  Clock/1 -> Sum1/1
  Sum1/1 -> Switch/2
  T1/1 -> [T1], To Workspace/1, "Time constant - open thruster "/1
  Divide2/1 -> Abs/1  "Maximum Time allowed"
  From2/1 -> Divide2/1
  From3/1 -> Divide2/2
  From4/1 -> Variable Time Delay/1
  Variable Time Delay/1 -> Goto2/1
  From5/1 -> Sum/2
  Abs/1 -> Variable Time Delay/2

== system Detumbling_using_engine_sim/Engine Model/If Action Subsystem2/If Action Subsystem Yaw -/thruster 2 ==
  T1 : Inport
  Abs : Abs  Commented=on  SaturateOnIntegerOverflow=off
  Divide2 : Product  Commented=on  Inputs=*/
  From2 : From  Commented=on  GotoTag=impulseBit_BiProp
  From3 : From  Commented=on  GotoTag=T2
  From4 : From  Commented=on  GotoTag=T2
  From5 : From  Commented=on  GotoTag=Stop_step
  Goto2 : Goto  Commented=on  GotoTag=Stop_step
  Initial Body Angular rates [deg/sec] : Constant  Value=Params.ImpulseBit_BiProp
  Scope : Scope
  Sum : Sum  Inputs=|+-
  "Time constant - open thruster " : TransferFcn  Denominator=[tau_Thrusters 1]
  To Workspace : ToWorkspace  Commented=on  VariableName=T1  SaveFormat=Timeseries  SampleTime=-1
  Variable Time Delay : VariableTransportDelay  Commented=on  MaximumDelay=50
  Thrust_2 : Outport
  wires:
  "Time constant - open thruster "/1 -> Sum/1
  Sum/1 -> Scope/1, Thrust_2/1
  Initial Body Angular rates [deg/sec]/1 -> [impulseBit_BiProp]
  T1/1 -> [T2], To Workspace/1, "Time constant - open thruster "/1
  From3/1 -> Divide2/2
  Divide2/1 -> Abs/1  "Maximum Time allowed"
  From4/1 -> Variable Time Delay/1
  Variable Time Delay/1 -> Goto2/1
  From2/1 -> Divide2/1
  From5/1 -> Sum/2
  Abs/1 -> Variable Time Delay/2

== system Detumbling_using_engine_sim/Engine Model/If Action Subsystem2/If Action Subsystem Yaw -/thruster 3 ==
  T1 : Inport
  Abs : Abs  Commented=on  SaturateOnIntegerOverflow=off
  Divide2 : Product  Commented=on  Inputs=*/
  From2 : From  Commented=on  GotoTag=impulseBit_BiProp
  From3 : From  Commented=on  GotoTag=T3
  From4 : From  Commented=on  GotoTag=T3
  From5 : From  Commented=on  GotoTag=Stop_step
  Goto2 : Goto  Commented=on  GotoTag=Stop_step
  Initial Body Angular rates [deg/sec] : Constant  Value=Params.ImpulseBit_BiProp
  Scope : Scope
  Sum : Sum  Inputs=|+-
  "Time constant - open thruster " : TransferFcn  Denominator=[tau_Thrusters 1]
  To Workspace : ToWorkspace  Commented=on  VariableName=T1  SaveFormat=Timeseries  SampleTime=-1
  Variable Time Delay1 : VariableTransportDelay  Commented=on  MaximumDelay=50
  Thrust_1 : Outport
  wires:
  "Time constant - open thruster "/1 -> Sum/1
  Sum/1 -> Scope/1, Thrust_1/1
  Initial Body Angular rates [deg/sec]/1 -> [impulseBit_BiProp]
  T1/1 -> [T3], To Workspace/1, "Time constant - open thruster "/1
  From3/1 -> Divide2/2
  Divide2/1 -> Abs/1  "Maximum Time allowed"
  From4/1 -> Variable Time Delay1/1
  Variable Time Delay1/1 -> Goto2/1
  From2/1 -> Divide2/1
  From5/1 -> Sum/2
  Abs/1 -> Variable Time Delay1/2

== system Detumbling_using_engine_sim/Engine Model/If Action Subsystem2/If Action Subsystem Yaw -/thruster 4  ==
  T1 : Inport
  w_t_2 : Inport  Port=2
  w_t_3 : Inport  Port=3
  dw/dt : Inport  Port=4
  Abs : Abs  Commented=on  SaturateOnIntegerOverflow=off
  Divide2 : Product  Commented=on  Inputs=*/
  From2 : From  Commented=on  GotoTag=impulseBit_BiProp
  From3 : From  Commented=on  GotoTag=T1
  From4 : From  Commented=on  GotoTag=T1
  From5 : From  Commented=on  GotoTag=Stop_step
  Goto2 : Goto  Commented=on  GotoTag=Stop_step
  Initial Body Angular rates [deg/sec] : Constant  Value=Params.ImpulseBit_BiProp
  Sum : Sum  Inputs=|+-
  "Time constant - open thruster " : TransferFcn  Denominator=[tau_Thrusters 1]
  To Workspace : ToWorkspace  Commented=on  VariableName=T1  SaveFormat=Timeseries  SampleTime=-1
  Variable Time Delay1 : VariableTransportDelay  Commented=on  MaximumDelay=50
  Thrust_4 : Outport
  wires:
  "Time constant - open thruster "/1 -> Sum/1
  Sum/1 -> Thrust_4/1
  Initial Body Angular rates [deg/sec]/1 -> [impulseBit_BiProp]
  T1/1 -> [T1], To Workspace/1, "Time constant - open thruster "/1
  From2/1 -> Divide2/1
  From3/1 -> Divide2/2
  Divide2/1 -> Abs/1  "Maximum Time allowed"
  From4/1 -> Variable Time Delay1/1
  Variable Time Delay1/1 -> Goto2/1
  From5/1 -> Sum/2
  Abs/1 -> Variable Time Delay1/2

== matlab function Detumbling_using_engine_sim/Satellite Bus/Satellite Kinematics/MATLAB Function1 ==
  data: q input; CHI_matrix output
function CHI_matrix = CHI(q)

CHI_matrix = [q(4),-q(3),q(2);...
              q(3),q(4),-q(1);...
              -q(2),q(1),q(4);...
             -q(1),-q(2),-q(3)];

== matlab function Detumbling_using_engine_sim/Reaction Wheels model/RW3/MATLAB Function ==
  data: Commanded_Torque input; Torque output; Stored_Angular input; torquebox_data input
function Torque = RW_Torque(Commanded_Torque,Stored_Angular,torquebox_data)
Torque = Allowed_torque(Commanded_Torque, Stored_Angular, torquebox_data);

== matlab function Detumbling_using_engine_sim/Reaction Wheels model/RW4/MATLAB Function ==
  data: Commanded_Torque input; Torque output; Stored_Angular input; torquebox_data input
function Torque = RW_Torque(Commanded_Torque,Stored_Angular,torquebox_data)
Torque = Allowed_torque(Commanded_Torque, Stored_Angular, torquebox_data);

== matlab function Detumbling_using_engine_sim/Engine Model/thruster2/MATLAB Function ==
  data: Commanded_Torque input; Torque output; Stored_Angular input; torquebox_data input
function Torque = RW_Torque(Commanded_Torque,Stored_Angular,torquebox_data)
Torque = Allowed_torque(Commanded_Torque, Stored_Angular, torquebox_data);

== matlab function Detumbling_using_engine_sim/Engine Model/thruster3/MATLAB Function ==
  data: Commanded_Torque input; Torque output; Stored_Angular input; torquebox_data input
function Torque = RW_Torque(Commanded_Torque,Stored_Angular,torquebox_data)
Torque = Allowed_torque(Commanded_Torque, Stored_Angular, torquebox_data);

== matlab function Detumbling_using_engine_sim/Engine Model/thruster4/MATLAB Function ==
  data: Commanded_Torque input; Torque output; Stored_Angular input; torquebox_data input
function Torque = RW_Torque(Commanded_Torque,Stored_Angular,torquebox_data)
Torque = Allowed_torque(Commanded_Torque, Stored_Angular, torquebox_data);

== matlab function Detumbling_using_engine_sim/Reaction Wheels model/RW2/MATLAB Function ==
  data: Commanded_Torque input; Torque output; Stored_Angular input; torquebox_data input
function Torque = RW_Torque(Commanded_Torque,Stored_Angular,torquebox_data)
Torque = Allowed_torque(Commanded_Torque, Stored_Angular, torquebox_data);
